simulink model "Simulink_rotacional"  (R2024a)
settings: Solver=VariableStepAuto  StartTime=0.0  StopTime=10.0  RelTol=1e-3
InitFcn:
  | m=10;
  | k=100;
  | r=0.05;

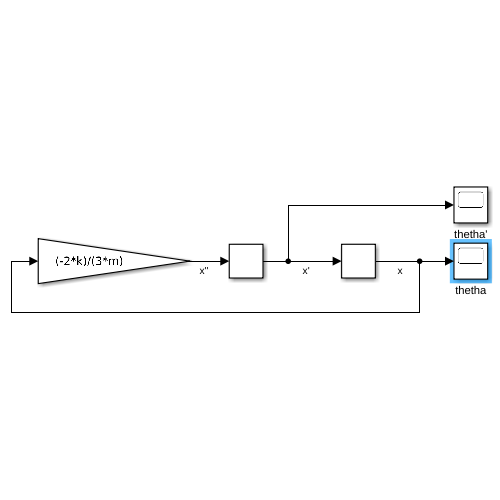
[thumbnail: Simulink's stored preview of the top-level diagram]
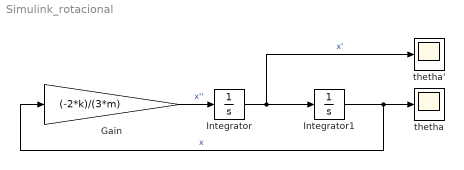
== system Simulink_rotacional ==
  Gain : Gain  Gain=(-2*k)/(3*m)
  Integrator : Integrator  InitialCondition=2
  Integrator1 : Integrator
  thetha : Scope
  thetha' : Scope
  wires:
  Integrator/1 -> thetha'/1, Integrator1/1  "x'"
  Gain/1 -> Integrator/1  "x''"
  Integrator1/1 -> Gain/1, thetha/1  "x"
